simulink model "CAN_Model_Rx"  (R2018b)
settings: Solver=VariableStepAuto  StartTime=0.0  StopTime=10.0  RelTol=1e-3
libraries: simulink_extras x1
settings Model: Creator=MAX_1  LastModifiedBy=MAX_1

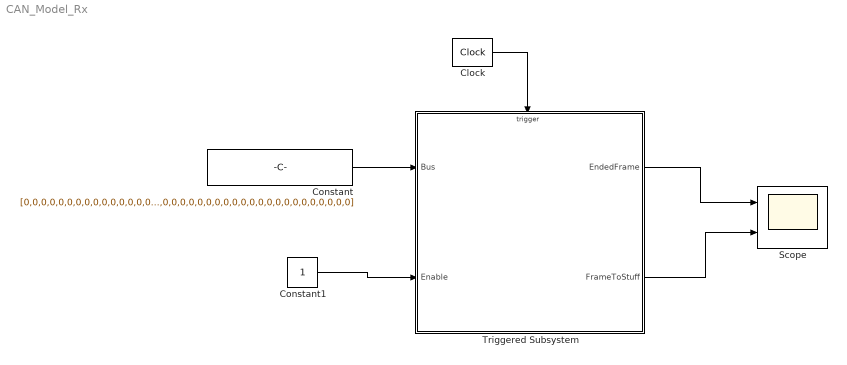
== system CAN_Model_Rx ==
  Clock : simulink_extras/Flip Flops/Clock  period=0.2
  Constant : Constant  Value=[0,0,0,0,0,0,0,0,0,0,0,0,0,0,0,0,0,0,0,0,0,0,0,0,0,0,0,0,0,0,0,0,0,0,0,0,0,0,0,0,0,0,0,0,0,0,0,0,0,0,0,0,0,0,0,0,0,0,0,0,0,0,0,0,0,0,0,0,0,0,0,0,0,0,0,0,0,0,0,0,0,0,0,0,0,0,0,0,0,0,0,0,0,0,0,0,0,0,0,0,0,0,0,0,0,0,0,0,0,0,0,0,0,0,0,0,0,0,0,0,0,0,0,0,0,0,0,0,0,0,0,0,0,0,0]
  Constant1 : Constant
  Scope : Scope  NumInputPorts=2
  Triggered Subsystem : Subsystem  TreatAsAtomicUnit=on
  wires:
  Constant/1 -> Triggered Subsystem/1(Bus)
  Constant1/1 -> Triggered Subsystem/2(Enable)
  Triggered Subsystem/2(FrameToStuff) -> Scope/2
  Triggered Subsystem/1(EndedFrame) -> Scope/1
  Clock/1 -> Triggered Subsystem/Trigger

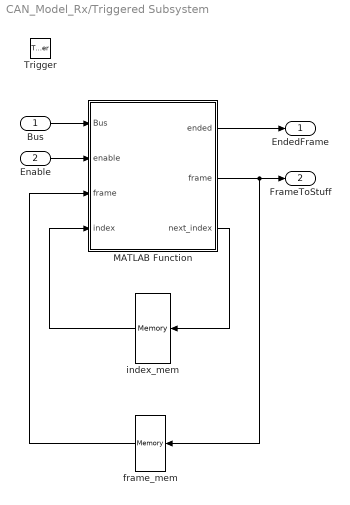
== system CAN_Model_Rx/Triggered Subsystem ==
  Bus : Inport
  Enable : Inport  Port=2
  Trigger : TriggerPort  VariantControl=Variant
  MATLAB Function : MATLAB Function  TreatAsAtomicUnit=on
  frame_mem : Memory  InitialCondition=[0,0,0,0,0,0,0,0,0,0,0,0,0,0,0,0,0,0,0,0,0,0,0,0,0,0,0,0,0,0,0,0,0,0,0,0,0,0,0,0,0,0,0,0,0,0,0,0,0,0,0,0,0,0,0,0,0,0,0,0,0,0,0,0,0,0,0,0,0,0,0,0,0,0,0,0,0,0,0,0,0,0,0,0,0,0,0,0,0,0,0,0,0,0,0,0,0,0,0,0,0,0,0,0,0,0,0,0,0,0,0,0,0,0,0,0,0,0,0,0,0,0,0,0,0,0,0,0,0,0,0,0,0,0,0]  InheritSampleTime=on
  index_mem : Memory  InitialCondition=135  InheritSampleTime=on
  EndedFrame : Outport
  FrameToStuff : Outport  Port=2
  wires:
  Enable/1 -> MATLAB Function/2(enable)
  Bus/1 -> MATLAB Function/1(Bus)
  MATLAB Function/3(next_index) -> index_mem/1
  frame_mem/1 -> MATLAB Function/3("frame ")
  MATLAB Function/1(ended) -> EndedFrame/1
  MATLAB Function/2(frame) -> frame_mem/1, FrameToStuff/1
  index_mem/1 -> MATLAB Function/4(index)

== matlab function CAN_Model_Rx/Triggered Subsystem/MATLAB Function ==
  data: ended output; Bus input; enable input; frame output; frame input; index input; next_index output
%riempio il frame a partire da 135 (la sua lunghezza) per avere già gli elementi
%in ordine giusto (ma con degli zeri in più all'inizio)
function [ended, frame, next_index] = readBus(Bus, enable, frame, index)
ended=0;
consecutive_ones=1;
consecutive_zeros=1;
if enable==1
    
    if index>=1 %praticamente sempre
        
        frame(index)=Bus;
        next_index=index-1;
        for i = length(frame)-index+1 : length(frame)-1
            if frame(i)==frame(i+1)
                if frame(i)==1
                    consecutive_ones=consecutive_ones+1;
                end
                if frame(i)==0
                    consecutive_zeros=consecutive_zeros+1;
                end
            end
            if frame(i)~=frame(i+1)
                consecutive_ones=0;
                consecutive_zeros=0;
            end

            if consecutive_ones==11
                ended=1;
                break;
            end
            if consecutive_zeros==7
                ended=2;
                break;
            end
        end
        if ended==1 || ended==2
            next_index=135;
        end
    else %non arrivo mai qui perché resetto l'indice già quando checkEOF==1 o ==2
        next_index=135; 
    end
    
end

end
